simulink model "PD_controller_for_FOIPTD_with_inner_SOIPTD_parametric"  (R2019b)
settings: Solver=ode45  StartTime=0.0  StopTime=30  MaxStep=1e-3  RelTol=1e-3  EnableMultiTasking=on
undefined symbols (not defined in the file or in its folder): D, D_inner, K, K_inner, P, P_inner, T1, T1_inner, T2_inner, tau, tau_inner
libraries: simulink x1
settings Model: Creator=msa  LastModifiedBy=aaa_b
settings DataIOCC: SaveFormat=Array  DSMLogging=off  ReturnWorkspaceOutputs=off
settings OptimizationCC: LifeSpan=inf
settings DebuggingCC: SolverPrmCheckMsg=warning  SFUnexpectedBacktrackingDiag=warning  SFNoUnconditionalDefaultTransitionDiag=warning  SFExecutionAtInitializationDiag=none  ArithmeticOperatorsInVariantConditions=warning
settings HardwareCC: ProdBitPerPointer=32  ProdBitPerSizeT=32  ProdBitPerPtrDiffT=32  ProdLargestAtomicFloat=None  ProdIntDivRoundTo=Undefined  ProdEndianess=Unspecified  ProdWordSize=32  ProdHWDeviceType=32-bit Generic
settings ModelReferenceCC: PropagateSignalLabelsOutOfModel=off
settings SFSimCC: SimUseLocalCustomCode=off  CustomCodeUndefinedFunction=UseInterfaceOnly
settings RTWCC: RTWUseLocalCustomCode=off
settings CodeAppCC: StateflowObjectComments=on
settings GRTTargetCC: TargetLangStandard=C89/C90 (ANSI)  GeneratePreprocessorConditionals=Disable all
settings ConfigComp: CovMetricSettings=dw  CovHtmlReporting=on  CovSaveCumulativeToWorkspaceVar=on  CovSaveSingleToWorkspaceVar=on  CovExternalEMLEnable=off  CovSFcnEnable=off

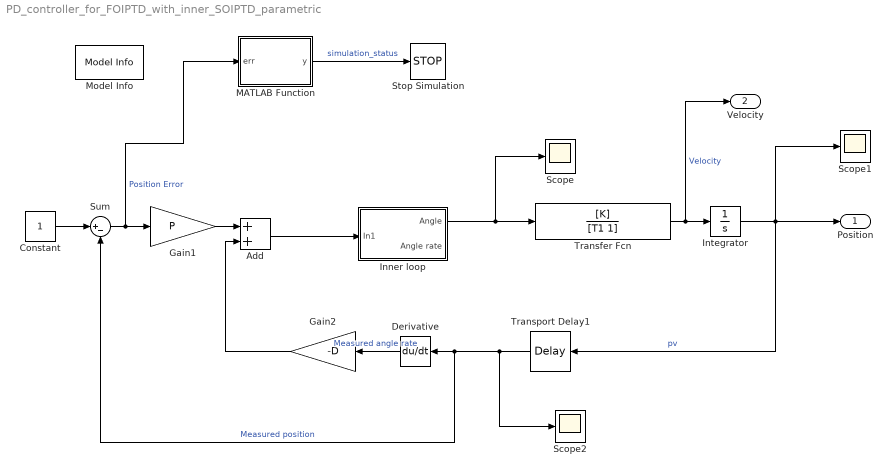
== system PD_controller_for_FOIPTD_with_inner_SOIPTD_parametric ==
  Add : Sum
  Constant : Constant
  Derivative : Derivative
  Gain1 : Gain  Gain=P
  Gain2 : Gain  Gain=-D
  "Inner loop " : Subsystem
  Integrator : Integrator
  MATLAB Function : MATLAB Function  TreatAsAtomicUnit=on
  Model Info : simulink/Model-Wide Utilities/Model Info  Frame=on  DisplayStringWithTags=Model Info How should we take sensors reading WITHOUT delay  HorizontalTextAlignment=Center  LeftAlignmentValue=0.5
  Scope : Scope
  Scope1 : Scope
  Scope2 : Scope
  Stop Simulation : Stop
  Sum : Sum  Inputs=|+-
  Transfer Fcn : TransferFcn  Numerator=[K]  Denominator=[T1 1]
  Transport Delay1 : TransportDelay  DelayTime=tau
  "Position " : Outport
  "Velocity " : Outport  Port=2
  wires:
  MATLAB Function/1(y) -> Stop Simulation/1  "simulation_status"
  "Inner loop "/1("Angle ") -> Scope/1, Transfer Fcn/1
  Gain2/1 -> Add/2
  Gain1/1 -> Add/1
  Constant/1 -> Sum/1
  Sum/1 -> MATLAB Function/1(err), Gain1/1  "Position Error"
  Transport Delay1/1 -> Scope2/1, Sum/2, Derivative/1  "Measured position"
  Integrator/1 -> Scope1/1, "Position "/1, Transport Delay1/1  "pv"
  Derivative/1 -> Gain2/1  "Measured angle rate"
  Transfer Fcn/1 -> "Velocity "/1, Integrator/1  "Velocity"
  Add/1 -> "Inner loop "/1(In1)

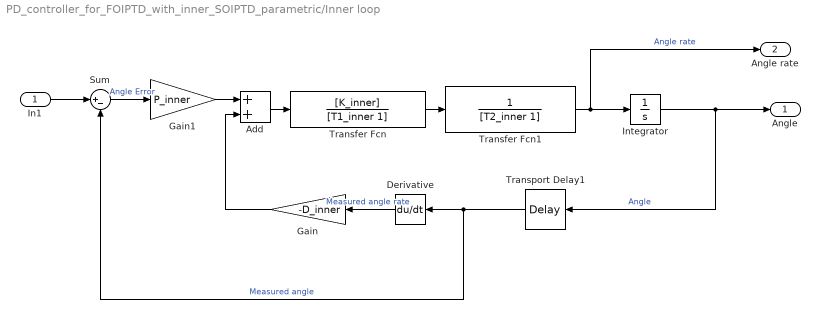
== system PD_controller_for_FOIPTD_with_inner_SOIPTD_parametric/Inner loop  ==
  In1 : Inport
  Add : Sum
  Derivative : Derivative
  Gain : Gain  Gain=-D_inner
  Gain1 : Gain  Gain=P_inner
  Integrator : Integrator
  Sum : Sum  Inputs=|+-
  Transfer Fcn : TransferFcn  Numerator=[K_inner]  Denominator=[T1_inner 1]
  Transfer Fcn1 : TransferFcn  Denominator=[T2_inner 1]
  Transport Delay1 : TransportDelay  DelayTime=tau_inner
  "Angle " : Outport
  "Angle rate " : Outport  Port=2
  wires:
  Sum/1 -> Gain1/1  "Angle Error"
  Transport Delay1/1 -> Sum/2, Derivative/1  "Measured angle"
  Transfer Fcn1/1 -> "Angle rate "/1, Integrator/1  "Angle rate"
  In1/1 -> Sum/1
  Transfer Fcn/1 -> Transfer Fcn1/1
  Gain1/1 -> Add/1
  Derivative/1 -> Gain/1  "Measured angle rate"
  Add/1 -> Transfer Fcn/1
  Gain/1 -> Add/2
  Integrator/1 -> Transport Delay1/1, "Angle "/1  "Angle"

== matlab function PD_controller_for_FOIPTD_with_inner_SOIPTD_parametric/MATLAB Function ==
  data: err input; y output
function y = fcn(err)
if (abs(err)>1000)
    y=1;
else
    y=0;
end
